simulink model "ControlSystemExercise3"  (R2019b)
settings: Solver=VariableStepAuto  StartTime=0.0  StopTime=10  RelTol=1e-6  AbsTol=1e-5
libraries: simulink x2
settings Model: Creator=19398  LastModifiedBy=19398

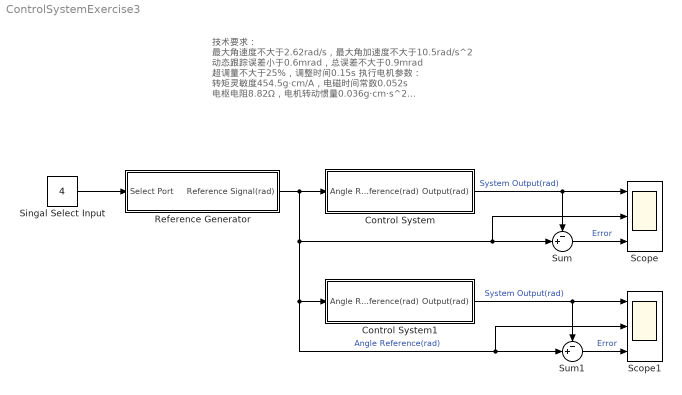
== system ControlSystemExercise3 ==
  note: 技术要求：
      | 最大角速度不大于2.62rad/s，最大角加速度不大于10.5rad/s^2
      | 动态跟踪误差小于0.6mrad，总误差不大于0.9mrad
      | 超调量不大于25%，调整时间0.15s
      | 执行电机参数：
      | 转矩灵敏度454.5g·cm/A，电磁时间常数0.052s
      | 电枢电阻8.82Ω，电机转动惯量0.036g·cm·s^2
      | 负载总转动惯量1000g·cm·s^2
  Control System : Subsystem
  Control System1 : Subsystem
  Reference Generator : Subsystem
  Scope : Scope  NumInputPorts=3
  Scope1 : Scope  NumInputPorts=3
  Singal Select Input : Constant  Value=4
  Sum : Sum  Inputs=-+|
  Sum1 : Sum  Inputs=-+|
  wires:
  Singal Select Input/1 -> Reference Generator/1(Select Port)
  Reference Generator/1(Reference Signal(rad)) -> Scope1/2, Sum1/2, Control System1/1(Angle Reference(rad)), Sum/2, Scope/2, Control System/1(Angle Reference(rad))  "Angle Reference(rad)"
  Control System/1(Output(rad)) -> Sum/1, Scope/1  "System Output(rad)"
  Sum/1 -> Scope/3  "Error"
  Control System1/1(Output(rad)) -> Sum1/1, Scope1/1  "System Output(rad)"
  Sum1/1 -> Scope1/3  "Error"

== system ControlSystemExercise3/Control System ==
  Angle Reference(rad) : Inport
  Angle Controller : Subsystem
  Control Voltage : Scope
  Mux : Mux  Inputs=2
  Plant : Subsystem
  Output(rad) : Outport
  wires:
  Angle Reference(rad)/1 -> Angle Controller/1(Angle Reference(rad))
  Angle Controller/1(Controller Output(V)) -> Control Voltage/1, Plant/1(Supply Voltage(V))
  Mux/1 -> Angle Controller/2(Feedback)  "Feedback"
  Plant/1(Angle(rad)) -> Mux/1, Output(rad)/1
  Plant/2(Angular Speed(rad/s)) -> Mux/2

== system ControlSystemExercise3/Control System1 ==
  Angle Reference(rad) : Inport
  Angle Controller : Subsystem
  Control Voltage(V) : Scope
  Plant : Subsystem
  Output(rad) : Outport
  wires:
  Angle Reference(rad)/1 -> Angle Controller/1(Angle Reference(rad))
  Angle Controller/1(Controller Output(V)) -> Control Voltage(V)/1, Plant/1(Supply Voltage(V))
  Plant/1(Angle(rad)) -> Output(rad)/1, Angle Controller/2(Angle Feedback(rad))  "Feedback"

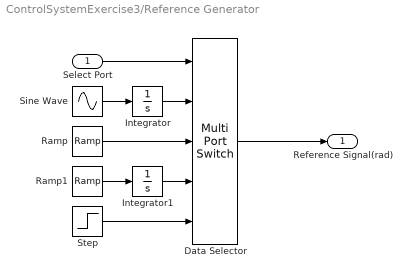
== system ControlSystemExercise3/Reference Generator ==
  Select Port : Inport
  Data Selector : MultiPortSwitch  Inputs=4
  Integrator : Integrator
  Integrator1 : Integrator
  Ramp : simulink/Sources/Ramp  slope=2.62  start=0  InitialOutput=0
  Ramp1 : simulink/Sources/Ramp  slope=10.5/2  start=0  InitialOutput=0
  Sine Wave : Sin  Amplitude=2.62  Frequency=10.5/2.62  SampleTime=0
  Step : Step  SampleTime=0
  Reference Signal(rad) : Outport
  wires:
  Select Port/1 -> Data Selector/1
  Data Selector/1 -> Reference Signal(rad)/1
  Sine Wave/1 -> Integrator/1
  Integrator/1 -> Data Selector/2
  Ramp/1 -> Data Selector/3
  Ramp1/1 -> Integrator1/1
  Integrator1/1 -> Data Selector/4
  Step/1 -> Data Selector/5

== system ControlSystemExercise3/Control System/Angle Controller ==
  Angle Reference(rad) : Inport
  Feedback : Inport  Port=2
  Angle Controller : Subsystem
  Angular Controller : Subsystem
  Demux : Demux  Outputs=2
  Controller Output(V) : Outport
  wires:
  Angle Reference(rad)/1 -> Angle Controller/1(Angle Reference(rad))  "Angle Reference(rad)"
  Feedback/1 -> Demux/1
  Demux/1 -> Angle Controller/2(Angle Feedback(rad))  "Angle Feedback(rad)"
  Demux/2 -> Angular Controller/2(Angular Speed Feedback(rad/s))  "Angular Feedback(rad/s)"
  Angular Controller/1(Angular Speed Controller Output(V)) -> Controller Output(V)/1
  Angle Controller/1(Angle Controller Output(rad/s)) -> Angular Controller/1(Angular Speed Reference(rad/s))  "Angular Speed Reference(rad/s)"

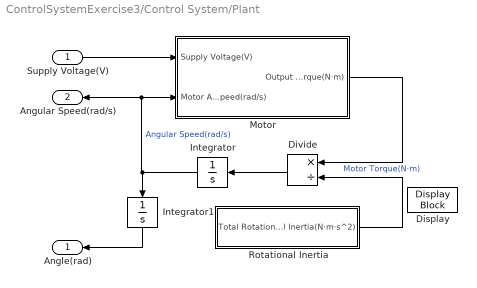
== system ControlSystemExercise3/Control System/Plant ==
  Supply Voltage(V) : Inport
  Display : DisplayBlock  LabelPosition=Hide  Format=short  Transparency=1
  Divide : Product  Inputs=*/
  Integrator : Integrator
  Integrator1 : Integrator
  Motor : Subsystem
  Rotational Inertia : Subsystem
  Angle(rad) : Outport
  Angular Speed(rad/s) : Outport  Port=2
  wires:
  Divide/1 -> Integrator/1
  Rotational Inertia/1(Total Rotational Inertia(N·m·s^2)) -> Divide/2
  Motor/1(Output Torque(N·m)) -> Divide/1  "Motor Torque(N·m)"
  Integrator/1 -> Angular Speed(rad/s)/1, Motor/2(Motor Angular Speed(rad/s)), Integrator1/1  "Angular Speed(rad/s)"
  Supply Voltage(V)/1 -> Motor/1(Supply Voltage(V))
  Integrator1/1 -> Angle(rad)/1

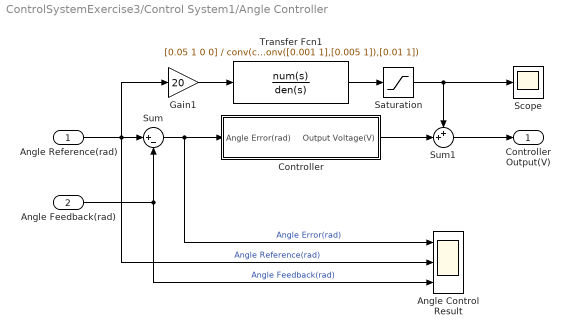
== system ControlSystemExercise3/Control System1/Angle Controller ==
  Angle Reference(rad) : Inport
  Angle Feedback(rad) : Inport  Port=2
  Angle Control Result : Scope  NumInputPorts=3
  Controller : Subsystem
  Gain1 : Gain  Gain=20
  Saturation : Saturate  UpperLimit=800  LowerLimit=-800
  Scope : Scope
  Sum : Sum  Inputs=|+-
  Sum1 : Sum  Inputs=++|
  Transfer Fcn1 : TransferFcn  Numerator=[0.05 1 0 0]  Denominator=conv(conv([0.001 1],[0.005 1]),[0.01 1])
  Controller Output(V) : Outport
  wires:
  Angle Reference(rad)/1 -> Gain1/1, Sum/1, Angle Control Result/2  "Angle Reference(rad)"
  Angle Feedback(rad)/1 -> Angle Control Result/3, Sum/2  "Angle Feedback(rad)"
  Sum/1 -> Controller/1(Angle Error(rad)), Angle Control Result/1  "Angle Error(rad)"
  Sum1/1 -> Controller Output(V)/1
  Transfer Fcn1/1 -> Saturation/1
  Gain1/1 -> Transfer Fcn1/1
  Controller/1(Output Voltage(V)) -> Sum1/2
  Saturation/1 -> Scope/1, Sum1/1

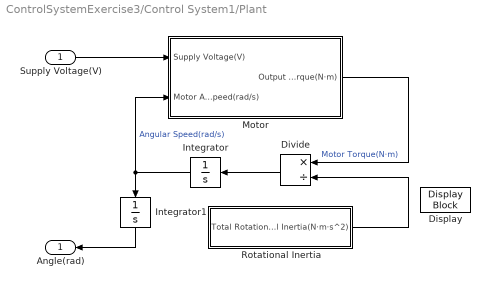
== system ControlSystemExercise3/Control System1/Plant ==
  Supply Voltage(V) : Inport
  Display : DisplayBlock  LabelPosition=Hide  Format=short  Transparency=1
  Divide : Product  Inputs=*/
  Integrator : Integrator
  Integrator1 : Integrator
  Motor : Subsystem
  Rotational Inertia : Subsystem
  Angle(rad) : Outport
  wires:
  Divide/1 -> Integrator/1
  Rotational Inertia/1(Total Rotational Inertia(N·m·s^2)) -> Divide/2
  Motor/1(Output Torque(N·m)) -> Divide/1  "Motor Torque(N·m)"
  Integrator/1 -> Motor/2(Motor Angular Speed(rad/s)), Integrator1/1  "Angular Speed(rad/s)"
  Integrator1/1 -> Angle(rad)/1
  Supply Voltage(V)/1 -> Motor/1(Supply Voltage(V))

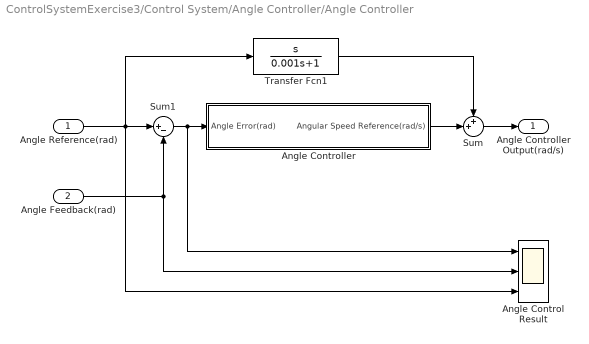
== system ControlSystemExercise3/Control System/Angle Controller/Angle Controller ==
  Angle Reference(rad) : Inport
  Angle Feedback(rad) : Inport  Port=2
  Angle Control Result : Scope  NumInputPorts=3
  Angle Controller : Subsystem
  Sum : Sum  Inputs=++|
  Sum1 : Sum  Inputs=|+-
  Transfer Fcn1 : TransferFcn  Numerator=[1 0]  Denominator=[0.001 1]
  Angle Controller Output(rad/s) : Outport
  wires:
  Transfer Fcn1/1 -> Sum/1
  Angle Reference(rad)/1 -> Sum1/1, Angle Control Result/3, Transfer Fcn1/1
  Sum/1 -> Angle Controller Output(rad/s)/1
  Angle Feedback(rad)/1 -> Angle Control Result/2, Sum1/2
  Sum1/1 -> Angle Controller/1(Angle Error(rad)), Angle Control Result/1
  Angle Controller/1(Angular Speed Reference(rad/s)) -> Sum/2

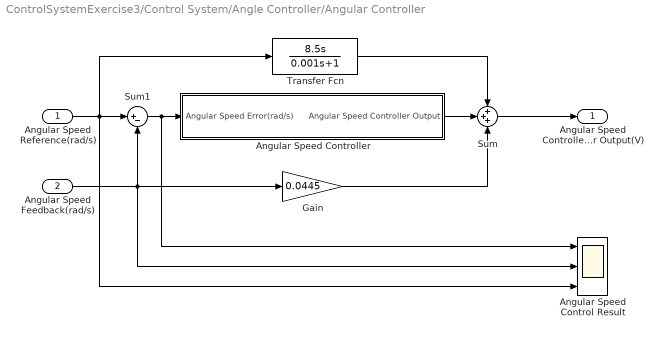
== system ControlSystemExercise3/Control System/Angle Controller/Angular Controller ==
  Angular Speed Reference(rad/s) : Inport
  Angular Speed Feedback(rad/s) : Inport  Port=2
  Angular Speed Control Result : Scope  NumInputPorts=3
  Angular Speed Controller : Subsystem
  Gain : Gain  Gain=0.0445
  Sum : Sum  Inputs=+++
  Sum1 : Sum  Inputs=|+-
  Transfer Fcn : TransferFcn  Numerator=[8.5 0]  Denominator=[0.001 1]
  Angular Speed Controller Output(V) : Outport
  wires:
  Transfer Fcn/1 -> Sum/1
  Angular Speed Reference(rad/s)/1 -> Transfer Fcn/1, Angular Speed Control Result/3, Sum1/1
  Sum/1 -> Angular Speed Controller Output(V)/1
  Angular Speed Feedback(rad/s)/1 -> Angular Speed Control Result/2, Gain/1, Sum1/2
  Sum1/1 -> Angular Speed Controller/1(Angular Speed Error(rad/s)), Angular Speed Control Result/1
  Angular Speed Controller/1(Angular Speed Controller Output) -> Sum/2
  Gain/1 -> Sum/3

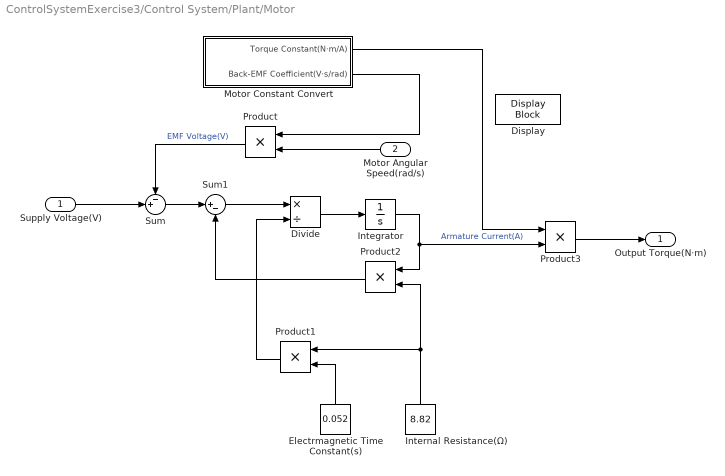
== system ControlSystemExercise3/Control System/Plant/Motor ==
  Supply Voltage(V) : Inport
  Motor Angular Speed(rad/s) : Inport  Port=2
  Display : DisplayBlock  LabelPosition=Hide  Format=short  Transparency=1
  Divide : Product  Inputs=*/
  Electrmagnetic Time Constant(s) : Constant  Value=0.052
  Integrator : Integrator
  Internal Resistance(Ω) : Constant  Value=8.82
  Motor Constant Convert : Subsystem
  Product{,1..3} (4 alike) : Product
  Sum : Sum  Inputs=-+|
  Sum1 : Sum  Inputs=|+-
  Output Torque(N·m) : Outport
  wires:
  Sum1/1 -> Divide/1
  Motor Constant Convert/2(Back-EMF Coefficient(V·s/rad)) -> Product/1
  Motor Angular Speed(rad/s)/1 -> Product/2
  Product2/1 -> Sum1/2
  Integrator/1 -> Product3/2, Product2/1  "Armature Current(A)"
  Product1/1 -> Divide/2
  Internal Resistance(Ω)/1 -> Product1/1, Product2/2
  Sum/1 -> Sum1/1
  Electrmagnetic Time Constant(s)/1 -> Product1/2
  Divide/1 -> Integrator/1
  Product3/1 -> Output Torque(N·m)/1
  Product/1 -> Sum/1  "EMF Voltage(V)"
  Motor Constant Convert/1(Torque Constant(N·m/A)) -> Product3/1
  Supply Voltage(V)/1 -> Sum/2

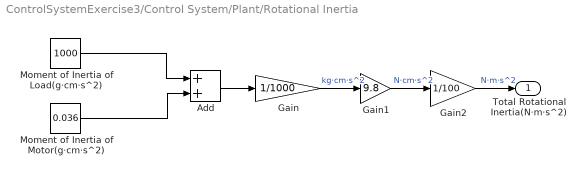
== system ControlSystemExercise3/Control System/Plant/Rotational Inertia ==
  Add : Sum
  Gain : Gain  Gain=1/1000
  Gain1 : Gain  Gain=9.8
  Gain2 : Gain  Gain=1/100
  Moment of Inertia of Load(g·cm·s^2) : Constant  Value=1000
  Moment of Inertia of Motor(g·cm·s^2) : Constant  Value=0.036
  Total Rotational Inertia(N·m·s^2) : Outport
  wires:
  Moment of Inertia of Load(g·cm·s^2)/1 -> Add/1
  Moment of Inertia of Motor(g·cm·s^2)/1 -> Add/2
  Add/1 -> Gain/1
  Gain/1 -> Gain1/1  "kg·cm·s^2"
  Gain1/1 -> Gain2/1  "N·cm·s^2"
  Gain2/1 -> Total Rotational Inertia(N·m·s^2)/1  "N·m·s^2"

== system ControlSystemExercise3/Control System1/Angle Controller/Controller ==
  Angle Error(rad) : Inport
  Gain : Gain  Gain=640
  Transfer Fcn : TransferFcn  Numerator=conv([0.05 1 0],[0.8 1])  Denominator=conv([1/114 1],[0.01 1 0])
  Output Voltage(V) : Outport
  wires:
  Angle Error(rad)/1 -> Gain/1
  Transfer Fcn/1 -> Output Voltage(V)/1
  Gain/1 -> Transfer Fcn/1

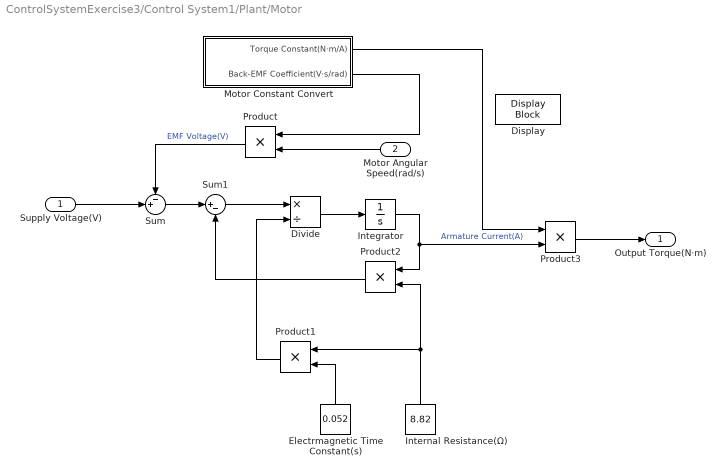
== system ControlSystemExercise3/Control System1/Plant/Motor ==
  Supply Voltage(V) : Inport
  Motor Angular Speed(rad/s) : Inport  Port=2
  Display : DisplayBlock  LabelPosition=Hide  Format=short  Transparency=1
  Divide : Product  Inputs=*/
  Electrmagnetic Time Constant(s) : Constant  Value=0.052
  Integrator : Integrator
  Internal Resistance(Ω) : Constant  Value=8.82
  Motor Constant Convert : Subsystem
  Product{,1..3} (4 alike) : Product
  Sum : Sum  Inputs=-+|
  Sum1 : Sum  Inputs=|+-
  Output Torque(N·m) : Outport
  wires:
  Sum1/1 -> Divide/1
  Motor Constant Convert/2(Back-EMF Coefficient(V·s/rad)) -> Product/1
  Motor Angular Speed(rad/s)/1 -> Product/2
  Product2/1 -> Sum1/2
  Integrator/1 -> Product3/2, Product2/1  "Armature Current(A)"
  Product1/1 -> Divide/2
  Internal Resistance(Ω)/1 -> Product1/1, Product2/2
  Sum/1 -> Sum1/1
  Electrmagnetic Time Constant(s)/1 -> Product1/2
  Divide/1 -> Integrator/1
  Product3/1 -> Output Torque(N·m)/1
  Product/1 -> Sum/1  "EMF Voltage(V)"
  Motor Constant Convert/1(Torque Constant(N·m/A)) -> Product3/1
  Supply Voltage(V)/1 -> Sum/2

== system ControlSystemExercise3/Control System1/Plant/Rotational Inertia ==
  Add : Sum
  Gain : Gain  Gain=1/1000
  Gain1 : Gain  Gain=9.8
  Gain2 : Gain  Gain=1/100
  Moment of Inertia of Load(g·cm·s^2) : Constant  Value=1000
  Moment of Inertia of Motor(g·cm·s^2) : Constant  Value=0.036
  Total Rotational Inertia(N·m·s^2) : Outport
  wires:
  Moment of Inertia of Load(g·cm·s^2)/1 -> Add/1
  Moment of Inertia of Motor(g·cm·s^2)/1 -> Add/2
  Add/1 -> Gain/1
  Gain/1 -> Gain1/1  "kg·cm·s^2"
  Gain1/1 -> Gain2/1  "N·cm·s^2"
  Gain2/1 -> Total Rotational Inertia(N·m·s^2)/1  "N·m·s^2"

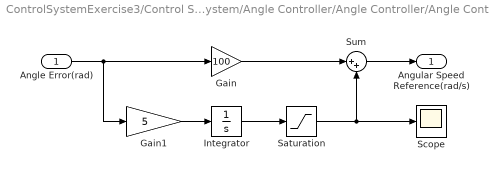
== system ControlSystemExercise3/Control System/Angle Controller/Angle Controller/Angle Controller ==
  Angle Error(rad) : Inport
  Gain : Gain  Gain=100
  Gain1 : Gain  Gain=5
  Integrator : Integrator
  Saturation : Saturate  UpperLimit=1  LowerLimit=-1
  Scope : Scope
  Sum : Sum  Inputs=|++
  Angular Speed Reference(rad/s) : Outport
  wires:
  Angle Error(rad)/1 -> Gain1/1, Gain/1
  Gain1/1 -> Integrator/1
  Integrator/1 -> Saturation/1
  Gain/1 -> Sum/1
  Saturation/1 -> Scope/1, Sum/2
  Sum/1 -> Angular Speed Reference(rad/s)/1

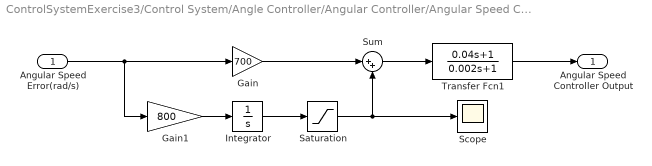
== system ControlSystemExercise3/Control System/Angle Controller/Angular Controller/Angular Speed Controller ==
  Angular Speed Error(rad/s) : Inport
  Gain : Gain  Gain=700
  Gain1 : Gain  Gain=800
  Integrator : Integrator
  Saturation : Saturate  UpperLimit=100  LowerLimit=-100
  Scope : Scope
  Sum : Sum  Inputs=|++
  Transfer Fcn1 : TransferFcn  Numerator=[0.04 1]  Denominator=[0.002 1]
  Angular Speed Controller Output : Outport
  wires:
  Angular Speed Error(rad/s)/1 -> Gain/1, Gain1/1
  Transfer Fcn1/1 -> Angular Speed Controller Output/1
  Sum/1 -> Transfer Fcn1/1
  Gain/1 -> Sum/1
  Integrator/1 -> Saturation/1
  Saturation/1 -> Scope/1, Sum/2
  Gain1/1 -> Integrator/1

== system ControlSystemExercise3/Control System/Plant/Motor/Motor Constant Convert ==
  Gain : Gain  Gain=1/1000
  Gain1 : Gain  Gain=9.8
  Gain2 : Gain  Gain=1/100
  Torque Sensitivity(g·cm/A) : Constant  Value=454.5
  Torque Constant(N·m/A) : Outport
  Back-EMF Coefficient(V·s/rad) : Outport  Port=2
  wires:
  Torque Sensitivity(g·cm/A)/1 -> Gain/1  "g·cm/A"
  Gain/1 -> Gain1/1  "kg·cm/A"
  Gain1/1 -> Gain2/1  "N·cm/A"
  Gain2/1 -> Back-EMF Coefficient(V·s/rad)/1, Torque Constant(N·m/A)/1  "N·m/A"

== system ControlSystemExercise3/Control System1/Plant/Motor/Motor Constant Convert ==
  Gain : Gain  Gain=1/1000
  Gain1 : Gain  Gain=9.8
  Gain2 : Gain  Gain=1/100
  Torque Sensitivity(g·cm/A) : Constant  Value=454.5
  Torque Constant(N·m/A) : Outport
  Back-EMF Coefficient(V·s/rad) : Outport  Port=2
  wires:
  Torque Sensitivity(g·cm/A)/1 -> Gain/1  "g·cm/A"
  Gain/1 -> Gain1/1  "kg·cm/A"
  Gain1/1 -> Gain2/1  "N·cm/A"
  Gain2/1 -> Back-EMF Coefficient(V·s/rad)/1, Torque Constant(N·m/A)/1  "N·m/A"
